simulink model "Didoumetry"  (R2021a)
settings: Solver=FixedStepAuto  StartTime=0.0  StopTime=inf  RelTol=1e-3
model workspace (MAT data in the model file):
  SL_ROS_VariableLengthArrays_MaxSizes.CommonInfo.ArrayTruncateAction = 'EmitWarning'
  SL_ROS_VariableLengthArrays_MaxSizes.MsgTypeMap = containers.Map
  SL_ROS_VariableLengthArrays_MaxSizes.MsgTypeMap.serialization.keys = {'sensor_msgs/CompressedImage'}
  SL_ROS_VariableLengthArrays_MaxSizes.MsgTypeMap.serialization.values{1}(1).PropertyName = 'Data'
  SL_ROS_VariableLengthArrays_MaxSizes.MsgTypeMap.serialization.values{1}(1).DataType = 'uint8'
  SL_ROS_VariableLengthArrays_MaxSizes.MsgTypeMap.serialization.values{1}(1).MaxLength = 198215
  SL_ROS_VariableLengthArrays_MaxSizes.MsgTypeMap.serialization.values{1}(2).PropertyName = 'Format'
  SL_ROS_VariableLengthArrays_MaxSizes.MsgTypeMap.serialization.values{1}(2).DataType = 'uint8'
  SL_ROS_VariableLengthArrays_MaxSizes.MsgTypeMap.serialization.values{1}(2).MaxLength = 128
  SL_ROS_VariableLengthArrays_MaxSizes.MsgTypeMap.serialization.uniformity = 0
  SL_ROS_VariableLengthArrays_MaxSizes.MsgTypeMap.serialization.keyType = 'char'
  SL_ROS_VariableLengthArrays_MaxSizes.MsgTypeMap.serialization.valueType = 'any'
libraries: robotlib x11
settings Model: SimulationMode=accelerator  EnablePacing=on  Creator=alexemdesgagne  LastModifiedBy=lamarre
settings SolverCC: AlgebraicLoopSolver=TrustRegion
settings OptimizationCC: EnhancedBackFolding=on  PassReuseOutputArgsAs=Individual arguments  ZeroExternalMemoryAtStartup=off  ZeroInternalMemoryAtStartup=off  MaxStackSize=64  OptimizeBlockOrder=speed  DifferentSizesBufferReuse=on  OptimizationCustomize=off  EfficientTunableParamExpr=on
settings DebuggingCC: ParameterTunabilityLossMsg=error  SFMachineParentedDataDiag=warning
settings HardwareCC: ProdBitPerPointer=32  ProdBitPerSizeT=32  ProdBitPerPtrDiffT=32  ProdLargestAtomicFloat=None  ProdIntDivRoundTo=Undefined  ProdEndianess=Unspecified  ProdWordSize=32  ProdHWDeviceType=Generic->Unspecified (assume 32-bit Generic)
settings SFSimCC: MATLABDynamicMemAlloc=off  SimTargetLang=C++
settings RTWCC: SystemTargetFile=ert.tlc  HardwareBoard=Robot Operating System (ROS)  TLCOptions="-aInlineSetEventsForThisBaseRateFcn=TLC_FALSE -aSuppressMultiTaskScheduler=TLC_FALSE  -aRateBasedStepFcn=0"  TemplateMakefile=ert_default_tmf  Toolchain=Catkin  TargetLang=C++
settings CodeAppCC: ForceParamTrailComments=on  IgnoreCustomStorageClasses=off  OperatorAnnotations=on  SimulinkDataObjDesc=on  SFDataObjDesc=on  InsertBlockDesc=on

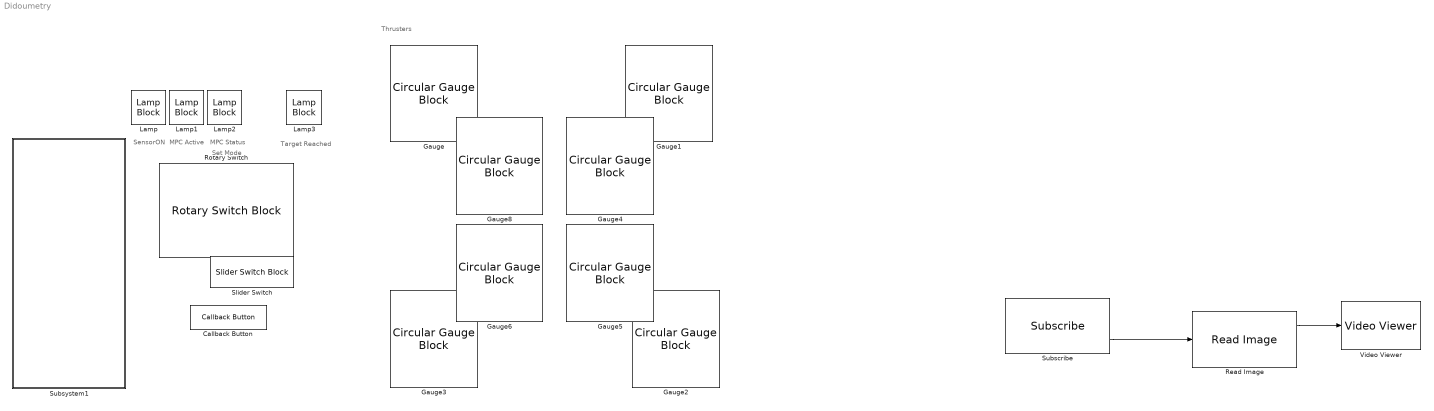
== system Didoumetry ==
  note: Thrusters
  note: Target Reached
  note: MPC Active
  note: SensorON
  note: MPC Status
  note: Set Mode
  Callback Button : CallbackButton  ButtonText=Dry Test
      settings: ClickFcn=sim('dry_test', 60);
  Gauge{,1..6,8} (8 alike) : CircularGaugeBlock  ScaleMin=-40  ScaleMax=50
  Lamp{,1..3} (4 alike) : LampBlock  LabelPosition=Hide
  Read Image : robotlib/Read Image  MaximumImageSize=[ 2500, 2500 ]  ImageEncoding=bgr8  ShowAlphaOutput=off  ShowErrorCodeOutput=on  VariableSizeOutputs=off
      settings: SourceProductBaseCode=RR
  Rotary Switch : RotarySwitchBlock  LabelPosition=Hide
      settings: Values={{'MPC AUTO', 'MPC 3DMouse', '3DMouse model', '3DMouse B matrix', 'Soft Kill', 'MPC Single Wpts'}, [10 19 20 21 0 11]}
  Slider Switch : SliderSwitchBlock
      settings: Values={{'Off', 'On'}, [0 1]}
  Subscribe : robotlib/Subscribe  topicSource=Select from ROS network  topic=/camera_array/cam0/image_raw/compressed  messageType=sensor_msgs/CompressedImage  SampleTime=-1  legacyBusStruct=off  messageQueueLength=1
  Subsystem1 : Subsystem
  Video Viewer : VideoViewer  FigPos=[68 1078 1853 942]
  wires:
  Subscribe/2 -> Read Image/1
  Read Image/1 -> Video Viewer/1

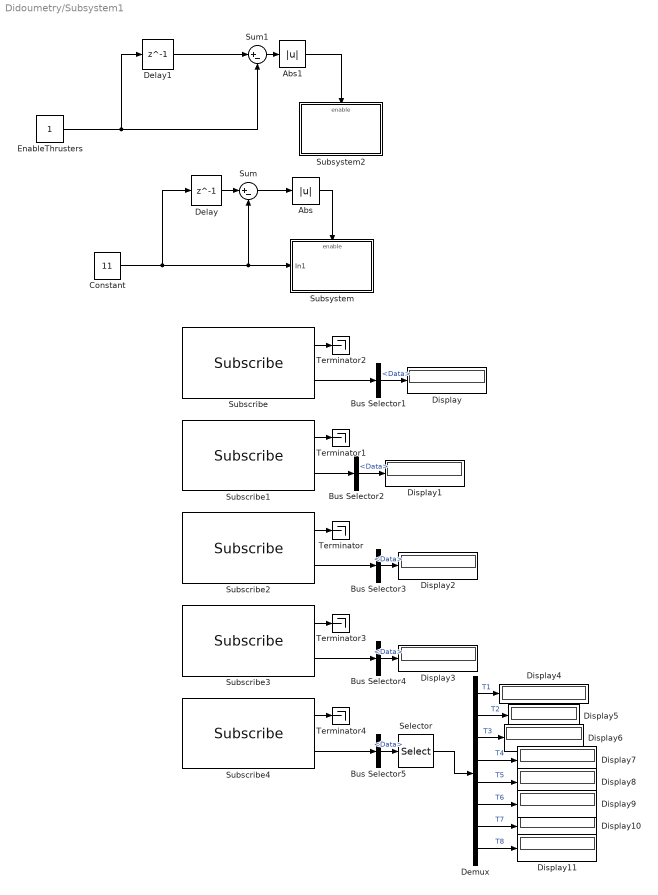
== system Didoumetry/Subsystem1 ==
  Abs : Abs
  Abs1 : Abs
  Bus Selector{1..5} (5 alike) : BusSelector  OutputSignals=Data
  Constant : Constant  Value=11
  Delay : Delay  DelayLength=1
  Delay1 : Delay  DelayLength=1
  Demux : Demux  Outputs=8
  Display{,1..11} (12 alike) : Display
  EnableThrusters : Constant
  Selector : Selector  InputPortWidth=128  IndexOptions=Index vector (dialog)  Indices=[1:8]  OutputSizes=1
  Subscribe : robotlib/Subscribe  topicSource=Select from ROS network  topic=/proc_control/sensor_on  messageType=std_msgs/Bool  SampleTime=-1  legacyBusStruct=off  messageQueueLength=1
  Subscribe1 : robotlib/Subscribe  topicSource=Select from ROS network  topic=/proc_control/is_mpc_active  messageType=std_msgs/Bool  SampleTime=-1  legacyBusStruct=off  messageQueueLength=1
  Subscribe2 : robotlib/Subscribe  topicSource=Select from ROS network  topic=/proc_control/mpc_status  messageType=std_msgs/Int8  SampleTime=-1  legacyBusStruct=off  messageQueueLength=1
  Subscribe3 : robotlib/Subscribe  topicSource=Select from ROS network  topic=/proc_control/target_reached  messageType=std_msgs/Bool  SampleTime=-1  legacyBusStruct=off  messageQueueLength=1
  Subscribe4 : robotlib/Subscribe  topicSource=Specify your own  topic=/telemetry/thruster_newton  messageType=std_msgs/Int8MultiArray  SampleTime=-1  legacyBusStruct=off  messageQueueLength=1
  Subsystem : Subsystem
  Subsystem2 : Subsystem
  Sum : Sum  Inputs=|+-
  Sum1 : Sum  Inputs=|+-
  Terminator{,1..4} (5 alike) : Terminator
  wires:
  Subscribe/2 -> Bus Selector1/1
  Subscribe1/1 -> Terminator1/1
  Delay/1 -> Sum/1
  Subscribe/1 -> Terminator2/1
  Subscribe2/1 -> Terminator/1
  Bus Selector1/1 -> Display/1  "<Data>"
  Constant/1 -> Delay/1, Sum/2, Subsystem/1(In1)
  Subscribe2/2 -> Bus Selector3/1
  Bus Selector3/1 -> Display2/1  "<Data>"
  Subscribe1/2 -> Bus Selector2/1
  Sum/1 -> Abs/1
  Bus Selector2/1 -> Display1/1  "<Data>"
  Abs/1 -> Subsystem/Enable
  Sum1/1 -> Abs1/1
  Delay1/1 -> Sum1/1
  Abs1/1 -> Subsystem2/Enable
  EnableThrusters/1 -> Sum1/2, Delay1/1
  Subscribe3/1 -> Terminator3/1
  Bus Selector4/1 -> Display3/1  "<Data>"
  Subscribe3/2 -> Bus Selector4/1
  Subscribe4/2 -> Bus Selector5/1
  Subscribe4/1 -> Terminator4/1
  Demux/1 -> Display4/1  "T1"
  Demux/2 -> Display5/1  "T2"
  Demux/3 -> Display6/1  "T3"
  Demux/4 -> Display7/1  "T4"
  Demux/5 -> Display8/1  "T5"
  Demux/6 -> Display9/1  "T6"
  Demux/7 -> Display10/1  "T7"
  Demux/8 -> Display11/1  "T8"
  Bus Selector5/1 -> Selector/1  "<Data>"
  Selector/1 -> Demux/1

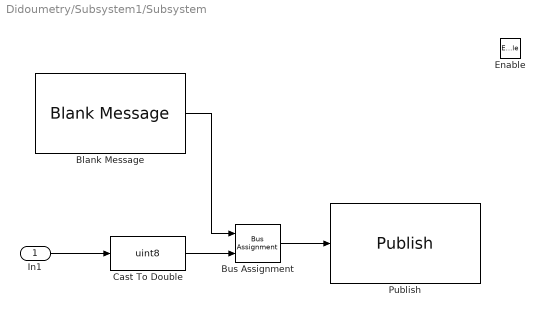
== system Didoumetry/Subsystem1/Subsystem ==
  In1 : Inport
  Enable : EnablePort
  Blank Message : robotlib/Blank Message  messageClass=Message  entityType=std_msgs/UInt8  messageType=std_msgs/UInt8  SampleTime=inf  legacyBusStruct=off
  Bus Assignment : BusAssignment  AssignedSignals=Data
  Cast To Double : DataTypeConversion  OutDataTypeStr=uint8
  Publish : robotlib/Publish  topicSource=Specify your own  topic=/proc_control/set_mode  messageType=std_msgs/UInt8  legacyBusStruct=off  messageQueueLength=1
  wires:
  Blank Message/1 -> Bus Assignment/1
  In1/1 -> Cast To Double/1
  Bus Assignment/1 -> Publish/1
  Cast To Double/1 -> Bus Assignment/2

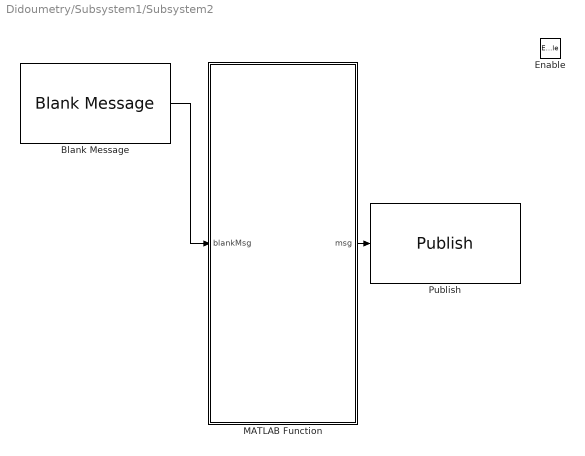
== system Didoumetry/Subsystem1/Subsystem2 ==
  Enable : EnablePort
  Blank Message : robotlib/Blank Message  messageClass=Message  entityType=sonia_common/ActivateAllPS  messageType=sonia_common/ActivateAllPS  SampleTime=inf  legacyBusStruct=off
  MATLAB Function : MATLAB Function  TreatAsAtomicUnit=on  SystemSampleTime=1/60
  Publish : robotlib/Publish  topicSource=Specify your own  topic=/provider_power/activate_all_ps  messageType=sonia_common/ActivateAllPS  legacyBusStruct=off  messageQueueLength=1
  wires:
  Blank Message/1 -> MATLAB Function/1(blankMsg)
  MATLAB Function/1(msg) -> Publish/1

== matlab function Didoumetry/Subsystem1/Subsystem2/MATLAB Function ==
  data: blankMsg input; msg output Bus: SL_Bus_Didoumetry_sonia_common_ActivateAllPS
function msg = assignEnableThrusters(blankMsg)
% assignStringInput - Assign a string a ROS message to specified input string
%
% MSG = assignStringInput(blankMsg, STR) assigns the input string, STR, to
%  a string field in the ROS message, blankMsg, and outputs the updated
%  ROS message.
%
%  Inputs
%    blankMsg: A bus for a 'std_msgs/String' message. This is 
%        used to initialize the output.
%    str: An array of uint8 that will be assigned to the 'Data' field
%        in blankMsg. The entire array is assumed to be a valid sequence of
%        character ASCII values.
% 
%  Outputs:
%    msg: A bus for a 'std_msgs/String' message, with the 'Data'
%        field set to a string.

%   Copyright 2015 The MathWorks, Inc.
%#codegen

% Note: The datatype of 'msg' has been explicitly set to the appropriate 
% Simulink bus type ("Bus: SL_Bus_robotROSMessageUsageExample_std_msgs_String"). 
%
% If the model name is changed, the datatype needs to be changed as well:
%   1) Click "Edit Data" in the Editor toolstrip to open "Ports and Data Manager"
%   2) Select "msg". From the "Type" dropdown, select "--- Refresh data types ---"
%   3) Set datatype to "Bus: SL_Bus_<modelname>_std_msgs_String"
   
msg = blankMsg;
msg.Slave = uint8(0);%uint8(49);
msg.Bus = uint8(0);
msg.Data = true;
